simulink model "rtwdemo_namerules"  (Simulink 7.6)
settings: Solver=FixedStepDiscrete  StartTime=0.0  StopTime=1  FixedStep=0.001  RelTol=1e-3
PreLoadFcn:
  | rtwdemo_namerules_data
values from neighbouring files (symbols this model uses):
  F1 = 2    [rtwdemo_dow_data.m]
  G1 = 4    [rtwdemo_dow_data.m]
  G2 = 5    [rtwdemo_dow_data.m]
  G3 = 6    [rtwdemo_dow_data.m]
  K1 = 3    [rtwdemo_cgv_init.m]    (also in rtwdemo_dow_data.m)
libraries: rtwdemowidgets x2
Description:
  | Applying Uniform Naming Conventions for Data Identifiers
settings Model: Creator=The MathWorks Inc.  ExtModeAutoUpdateStatusClock=off
settings MATStruct: SampleTime=0.001  Offset=0  Priority=[20.0]
settings DataIOCC: SaveOutput=off  SaveTime=off
settings OptimizationCC: InlineParams=on  InlineInvariantSignals=on  PassReuseOutputArgsAs=Individual arguments  StateBitsets=on  DataBitsets=on  UseTempVars=on  ZeroExternalMemoryAtStartup=off  ZeroInternalMemoryAtStartup=off  NoFixptDivByZeroProtection=on  EfficientFloat2IntCast=on  EfficientMapNaN2IntZero=off  OptimizeModelRefInitCode=on  LifeSpan=1  BufferReusableBoundary=off
settings DebuggingCC: CheckExecutionContextPreStartOutputMsg=on  CheckExecutionContextRuntimeOutputMsg=on  StrictBusMsg=ErrorOnBusTreatedAsVector
settings HardwareCC: ProdIntDivRoundTo=Zero  ProdEndianess=LittleEndian  ProdHWDeviceType=Generic->32-bit Embedded Processor  TargetHWDeviceType=Generic->32-bit Embedded Processor
settings SFSimCC: SimParseCustomCode=off
settings RTWCC: SystemTargetFile=ert.tlc  TemplateMakefile=ert_default_tmf  Description=Real-Time Workshop Embedded Coder (no auto configuration)  GenerateReport=on  RTWVerbose=off  ProcessScript=ert_make_rtw_hook  IncludeHyperlinkInReport=on  LaunchReport=on
settings CodeAppCC: ForceParamTrailComments=on  IgnoreCustomStorageClasses=off  IgnoreTestpoints=on  SimulinkDataObjDesc=on  CustomSymbolStrFcn=$N$M$F  CustomSymbolStrMacro=$N$M  DefineNamingRule=LowerCase  ParamNamingRule=LowerCase  SignalNamingRule=LowerCase  InsertBlockDesc=on
settings ERTTargetCC: TargetFcnLib=ansi_tfl_tmw.mat  MultiwordLength=2048  GenerateSampleERTMain=on  IncludeMdlTerminateFcn=off  SupportNonFinite=off  SupportComplex=off  InlinedParameterPlacement=NonHierarchical  ERTCustomFileTemplate=example_file_process.tlc  ConvertIfToSwitch=off

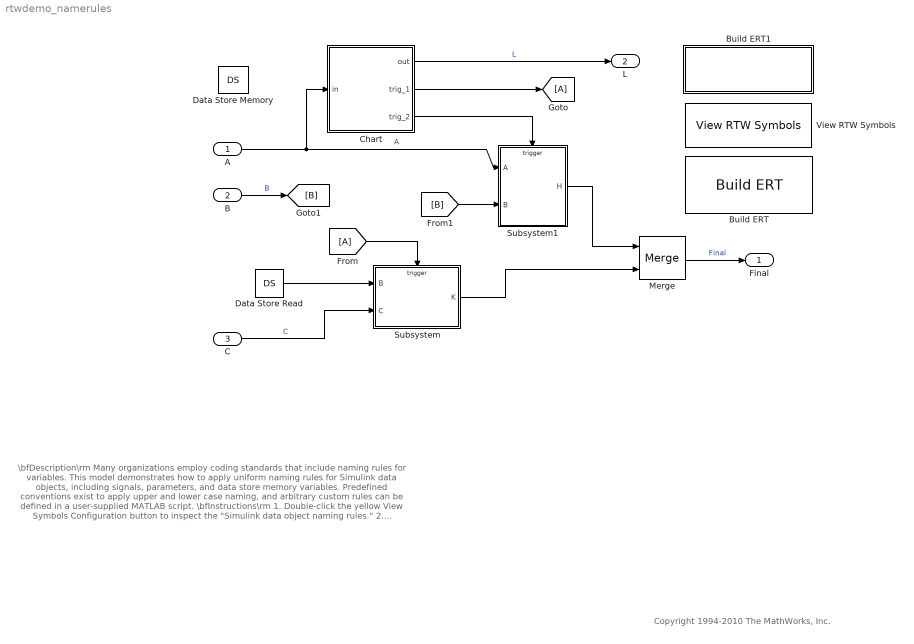
== system rtwdemo_namerules ==
  note: \bfDescription\rm
      | Many organizations employ coding standards that include naming rules for variables.  This model demonstrates
      | how to apply uniform naming rules for Simulink data objects, including signals, parameters, and data store memory
      | variables.  Predefined conventions exist to apply upper and lower case naming, and arbitrary custom rules can be
      | defined in a user-supplied MATLAB script.
      |
      | \bfInstructions\rm
      | 1. Double-click the yellow View Symbols Configuration button to inspect the "Simulink data object naming rules."
      | 2. Double-click the yellow Inspect Data Objects button to inspect the data objects for this model.
      | 3. Generate code using the blue button in the upper right of the diagram.  An HTML report automatically appears.
      | 4. Inspect the data that is defined toward the top of rtwdemo\_namerules.c.
      |
      | \bfNote\rm
      | The model is configured to "Force lower case."  Therefore, the variables in the code are defined in lower case
      | even though the data is declared upper case in the model.
  note: Copyright 1994-2010 The MathWorks, Inc.
  A : Inport  OutDataTypeStr=double  PortDimensions=1  SampleTime=0.001
  B : Inport  Port=2  OutDataTypeStr=double  PortDimensions=1  SampleTime=0.001
  C : Inport  Port=3  OutDataTypeStr=double  PortDimensions=1  SampleTime=0.001
  Build ERT : rtwdemowidgets/Build ERT  SystemSampleTime=-1  attrib_overrides={}
  Build ERT1 : Subsystem  mask{attrib_overrides={}}
      mask prompts: attrib_overrides "List of attributes to preserve (cell of strings):"
      mask help: Invoke Model Explorer
      settings: OpenFcn=rtwprivate daexplrwsview;
      mask Display:
      | disp(['Inspect Data Objects\n',...
      | 	  '(double-click)'])
  Chart : Stateflow chart  TreatAsAtomicUnit=on  RTWFcnName=entry_point  RTWFileName=sfcc
      settings: RTWFcnNameOpts=User specified
  Data Store Memory : DataStoreMemory  DataStoreName=DS
  Data Store Read : DataStoreRead  DataStoreName=DS  SampleTime=0.001
  Merge : Merge
  Subsystem : Subsystem  TreatAsAtomicUnit=on
  Subsystem1 : Subsystem  TreatAsAtomicUnit=on
  View RTW Symbols : rtwdemowidgets/View RTW Symbols  SystemSampleTime=-1
  Final : Outport
  L : Outport  Port=2
  wires:
  C/1 -> Subsystem/2(C)  "C"
  A/1 -> Subsystem1/1(A), Chart/1(in)  "A"
  Subsystem1/1(H) -> Merge/1
  Subsystem/1(K) -> Merge/2
  Merge/1 -> Final/1  "Final"
  Chart/3(trig_2) -> Subsystem1/Trigger
  Chart/2(trig_1) -> [A]
  [A] -> Subsystem/Trigger
  Chart/1(out) -> L/1  "L"
  B/1 -> [B]  "B"
  [B] -> Subsystem1/2(B)
  Data Store Read/1 -> Subsystem/1(B)

== system rtwdemo_namerules/Build ERT1 ==

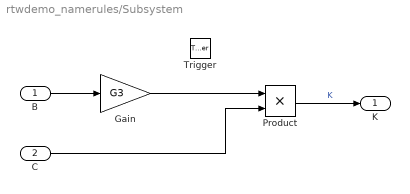
== system rtwdemo_namerules/Subsystem ==
  B : Inport
  C : Inport  Port=2
  Trigger : TriggerPort  TriggerType=function-call
  Gain : Gain  Gain=G3
  Product : Product  RndMeth=Zero
  K : Outport
  wires:
  B/1 -> Gain/1
  Gain/1 -> Product/1
  C/1 -> Product/2
  Product/1 -> K/1  "K"

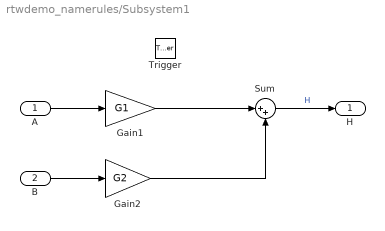
== system rtwdemo_namerules/Subsystem1 ==
  A : Inport
  B : Inport  Port=2
  Trigger : TriggerPort  TriggerType=function-call
  Gain1 : Gain  Gain=G1
  Gain2 : Gain  Gain=G2
  Sum : Sum  Inputs=|++
  H : Outport
  wires:
  A/1 -> Gain1/1
  Gain1/1 -> Sum/1
  B/1 -> Gain2/1
  Gain2/1 -> Sum/2
  Sum/1 -> H/1  "H"

== stateflow chart Chart ==
  (default) -> (junction 3)
  (junction 3) -> (junction 4) [order 2] : {
      |   out = in;
      |   trig_2;
      | }
  (junction 3) -> (junction 4) [order 1] : [F1 > 10]
      | {
      |   out = in * K1 * G1;
      |   trig_1;
      | }
  data: K1 parameter double; G1 parameter double; in input double; out output double; F1 parameter double
  events: trig_1 output FUNCTION_CALL_EVENT; trig_2 output FUNCTION_CALL_EVENT
